simulink model "ConnectionControl"  (R2024b)
settings: Solver=VariableStepAuto  StartTime=0.0  StopTime=10.0  RelTol=1e-3
libraries: spsIdealSwitchLib x6
settings Model: Creator=Korisnik  LastModifiedBy=Korisnik

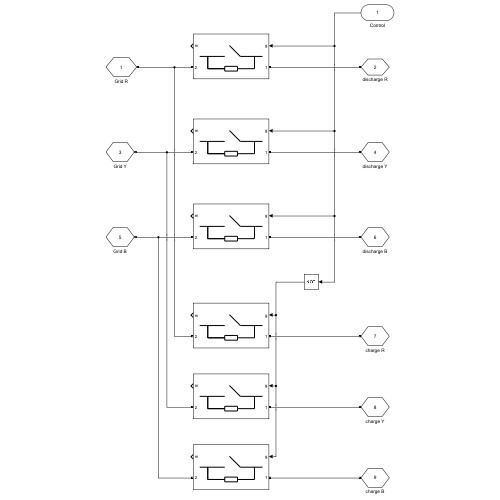
[thumbnail: Simulink's stored preview of the top-level diagram]
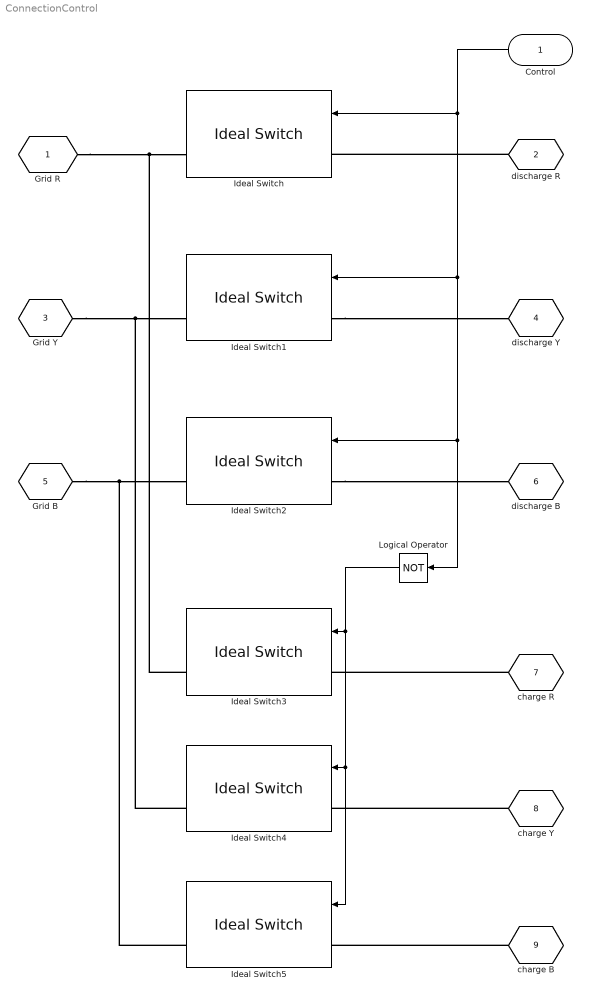
== system ConnectionControl ==
  Control : Inport
  Ideal Switch{,1..5} (6 alike) : spsIdealSwitchLib/Ideal Switch  Ron=0.001  Lon=0  IC=0  Rs=1e5  Cs=inf  Measurements=on
  Logical Operator : Logic  Operator=NOT  AllPortsSameDT=off  OutDataTypeStr=boolean
  Grid R : PMIOPort  Side=Left
  discharge R : PMIOPort  Port=2  Side=Right
  Grid Y : PMIOPort  Port=3  Side=Left
  discharge Y : PMIOPort  Port=4  Side=Left
  Grid B : PMIOPort  Port=5  Side=Left
  discharge B : PMIOPort  Port=6  Side=Left
  charge R : PMIOPort  Port=7  Side=Left
  charge Y : PMIOPort  Port=8  Side=Left
  charge B : PMIOPort  Port=9  Side=Left
  wires:
  Control/1 -> Logical Operator/1, Ideal Switch2/1, Ideal Switch1/1, Ideal Switch/1
  Logical Operator/1 -> Ideal Switch5/1, Ideal Switch4/1, Ideal Switch3/1
  connections:
  Grid R/RConn1 -- Ideal Switch3/RConn1 -- Ideal Switch/RConn1
  discharge R/RConn1 -- Ideal Switch/LConn1
  Ideal Switch1/LConn1 -- discharge Y/RConn1
  Grid Y/RConn1 -- Ideal Switch4/RConn1 -- Ideal Switch1/RConn1
  Grid B/RConn1 -- Ideal Switch5/RConn1 -- Ideal Switch2/RConn1
  Ideal Switch2/LConn1 -- discharge B/RConn1
  charge R/RConn1 -- Ideal Switch3/LConn1
  charge Y/RConn1 -- Ideal Switch4/LConn1
  charge B/RConn1 -- Ideal Switch5/LConn1
